simulink library "PhD_Library"  (R2018a)
settings: Solver=VariableStepAuto  StartTime=0.0  StopTime=10.0  RelTol=1e-3
values from neighbouring files (symbols this model uses):
  fn = 60    [Basics_01_Param.m]    (also in FIRs.m = 50; PostSubmission_FreqResp_00_Param.m; XoverRCalc.m)
  Ts_control = 1/20000    (= 5e-05)    [Basics_01_Param.m]    (also in PostSubmission_FreqResp_00_Param.m)
  Ts_PWM = 1/200000    (= 5e-06)    [Basics_01_Param.m]    (also in PostSubmission_FreqResp_00_Param.m)
  Uanp = 1    [Basics_01_Param.m]    (also in PostSubmission_FreqResp_00_Param.m)
undefined symbols (not defined in the file or in its folder): D1, Delta, DiscIntNeverNeededParam, ESS, Iap, PCC, Sn, tctrl, WT
libraries: $bdroot x49, powerlib_meascontrol x39, peTransforms x28, powerlib x18
(part 2 of 3)

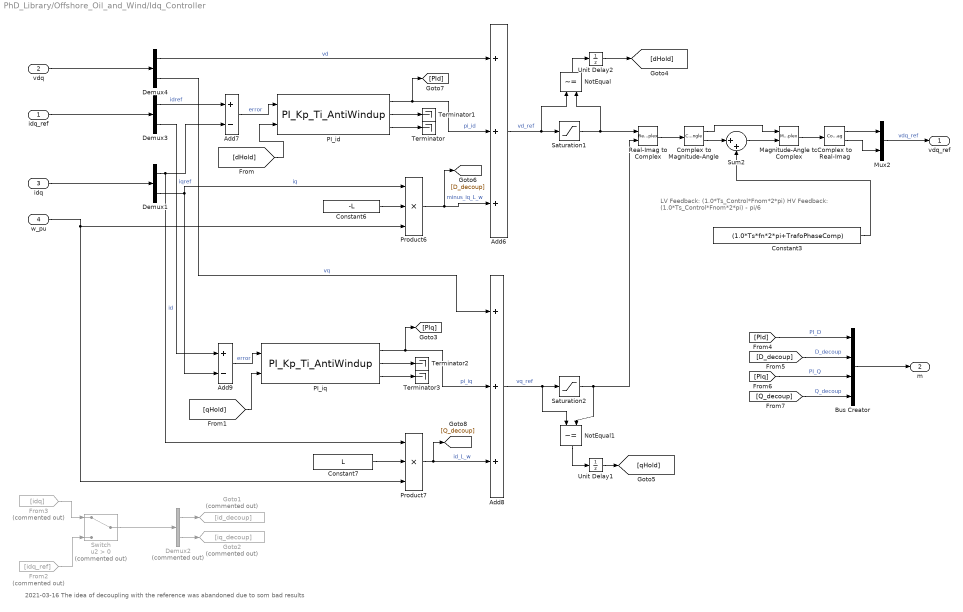
== system PhD_Library/Offshore_Oil_and_Wind/Idq_Controller ==
  note: LV Feedback: (1.0*Ts_Control*Fnom*2*pi)
      | HV Feedback: (1.0*Ts_Control*Fnom*2*pi) - pi/6
  note: 2021-03-16 The idea of decoupling with the reference was abandoned due to som bad results
  idq_ref : Inport
  vdq : Inport  Port=2
  idq : Inport  Port=3
  w_pu : Inport  Port=4
  Add6 : Sum  Inputs=+++
  Add7 : Sum  Inputs=+-
  Add8 : Sum  Inputs=+++
  Add9 : Sum  Inputs=+-
  Bus Creator : BusCreator  Inputs=4
  Complex to Magnitude-Angle : ComplexToMagnitudeAngle
  Complex to Real-Imag : ComplexToRealImag
  Constant3 : Constant  Value=(1.0*Ts*fn*2*pi+TrafoPhaseComp)  SampleTime=Ts
  Constant6 : Constant  Value=-L  SampleTime=Ts_control
  Constant7 : Constant  Value=L  SampleTime=Ts_control
  Demux1 : Demux  Outputs=2
  Demux2 : Demux  Commented=on  Outputs=2
  Demux3 : Demux  Outputs=2
  Demux4 : Demux  Outputs=2
  From2 : From  Commented=on  GotoTag=idq_ref
  From3 : From  Commented=on  GotoTag=idq
  Goto1 : Goto  Commented=on  GotoTag=id_decoup
  Goto2 : Goto  Commented=on  GotoTag=iq_decoup
  Magnitude-Angle to Complex : MagnitudeAngleToComplex
  Mux2 : Mux  Inputs=2
  NotEqual : RelationalOperator  Operator=~=  OutDataTypeStr=boolean  RndMeth=Simplest
  NotEqual1 : RelationalOperator  Operator=~=  OutDataTypeStr=boolean  RndMeth=Simplest
  PI_id : $bdroot/Offshore_Oil_and_Wind/PI_Kp_Ti_AntiWindup  Ts=Ts  Kp=Kp  Ti=Ti  I_ini=I_ini_d  PI_max=PI_max  PI_min=PI_min
  PI_iq : $bdroot/Offshore_Oil_and_Wind/PI_Kp_Ti_AntiWindup  Ts=Ts  Kp=Kp  Ti=Ti  I_ini=I_ini_q  PI_max=PI_max  PI_min=PI_min
  Product6 : Product  Inputs=3  RndMeth=Zero
  Product7 : Product  Inputs=3  RndMeth=Zero
  Real-Imag to Complex : RealImagToComplex
  Saturation1 : Saturate  UpperLimit=PI_max  LowerLimit=PI_min
  Saturation2 : Saturate  UpperLimit=PI_max  LowerLimit=PI_min
  Sum2 : Sum  Inputs=|++
  Switch : Switch  Commented=on  Criteria=u2 > Threshold
  Terminator{,1..3} (4 alike) : Terminator
  Unit Delay1 : UnitDelay  SampleTime=Ts
  Unit Delay2 : UnitDelay  SampleTime=Ts
  vdq_ref : Outport
  m : Outport  Port=2
  wires:
  PI_iq/1 -> [PIq], Add8/2  "pi_iq"
  PI_iq/2 -> Terminator2/1
  PI_id/2 -> Terminator1/1
  w_pu/1 -> Product7/3, Product6/3
  Add9/1 -> PI_iq/1  "error"
  PI_id/1 -> [PId], Add6/2  "pi_id"
  Constant6/1 -> Product6/2
  Constant7/1 -> Product7/2
  Demux1/1 -> Add7/2, Product7/1  "id"
  Product7/1 -> [Q_decoup], Add8/3  "id_L_w"
  Demux4/1 -> Add6/1  "vd"
  Add7/1 -> PI_id/1  "error"
  Demux1/2 -> Product6/1, Add9/2  "iq"
  Product6/1 -> [D_decoup], Add6/3  "minus_iq_L_w"
  PI_iq/3 -> Terminator3/1
  PI_id/3 -> Terminator/1
  Demux4/2 -> Add8/1  "vq"
  Mux2/1 -> vdq_ref/1  "vdq_ref"
  idq/1 -> Demux1/1
  vdq/1 -> Demux4/1
  Add8/1 -> NotEqual1/1, Saturation2/1  "vq_ref"
  Add6/1 -> NotEqual/1, Saturation1/1  "vd_ref"
  Demux2/1 -> Goto1/1
  Demux2/2 -> Goto2/1
  idq_ref/1 -> Demux3/1
  Demux3/1 -> Add7/1  "idref"
  Demux3/2 -> Add9/1  "iqref"
  Switch/1 -> Demux2/1
  From2/1 -> Switch/3
  From3/1 -> Switch/1
  Magnitude-Angle to Complex/1 -> Complex to Real-Imag/1
  Real-Imag to Complex/1 -> Complex to Magnitude-Angle/1
  Complex to Magnitude-Angle/1 -> Magnitude-Angle to Complex/1
  Complex to Magnitude-Angle/2 -> Sum2/1
  Sum2/1 -> Magnitude-Angle to Complex/2
  Constant3/1 -> Sum2/2
  Complex to Real-Imag/1 -> Mux2/1
  Complex to Real-Imag/2 -> Mux2/2
  [PId] -> Bus Creator/1  "PI_D"
  [D_decoup] -> Bus Creator/2  "D_decoup"
  [PIq] -> Bus Creator/3  "PI_Q"
  Bus Creator/1 -> m/1
  [Q_decoup] -> Bus Creator/4  "Q_decoup"
  Saturation1/1 -> NotEqual/2, Real-Imag to Complex/1
  NotEqual/1 -> Unit Delay2/1
  Saturation2/1 -> NotEqual1/2, Real-Imag to Complex/2
  NotEqual1/1 -> Unit Delay1/1
  Unit Delay2/1 -> [dHold]
  Unit Delay1/1 -> [qHold]
  [dHold] -> PI_id/2
  [qHold] -> PI_iq/2

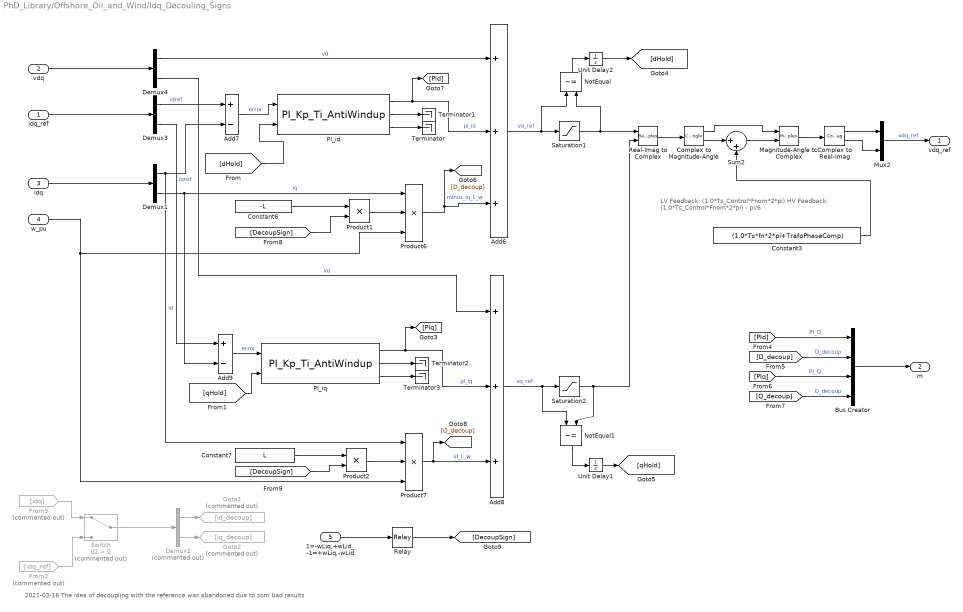
== system PhD_Library/Offshore_Oil_and_Wind/Idq_Decouling_Signs ==
  note: LV Feedback: (1.0*Ts_Control*Fnom*2*pi)
      | HV Feedback: (1.0*Ts_Control*Fnom*2*pi) - pi/6
  note: 2021-03-16 The idea of decoupling with the reference was abandoned due to som bad results
  idq_ref : Inport
  vdq : Inport  Port=2
  idq : Inport  Port=3
  w_pu : Inport  Port=4
  1=-wLiq,+wLid_-1=+wLiq,-wLid : Inport  Port=5
  Add6 : Sum  Inputs=+++
  Add7 : Sum  Inputs=+-
  Add8 : Sum  Inputs=+++
  Add9 : Sum  Inputs=+-
  Bus Creator : BusCreator  Inputs=4
  Complex to Magnitude-Angle : ComplexToMagnitudeAngle
  Complex to Real-Imag : ComplexToRealImag
  Constant3 : Constant  Value=(1.0*Ts*fn*2*pi+TrafoPhaseComp)  SampleTime=Ts
  Constant6 : Constant  Value=-L  SampleTime=Ts_control
  Constant7 : Constant  Value=L  SampleTime=Ts_control
  Demux1 : Demux  Outputs=2
  Demux2 : Demux  Commented=on  Outputs=2
  Demux3 : Demux  Outputs=2
  Demux4 : Demux  Outputs=2
  From2 : From  Commented=on  GotoTag=idq_ref
  From3 : From  Commented=on  GotoTag=idq
  Goto1 : Goto  Commented=on  GotoTag=id_decoup
  Goto2 : Goto  Commented=on  GotoTag=iq_decoup
  Magnitude-Angle to Complex : MagnitudeAngleToComplex
  Mux2 : Mux  Inputs=2
  NotEqual : RelationalOperator  Operator=~=  OutDataTypeStr=boolean  RndMeth=Simplest
  NotEqual1 : RelationalOperator  Operator=~=  OutDataTypeStr=boolean  RndMeth=Simplest
  PI_id : $bdroot/Offshore_Oil_and_Wind/PI_Kp_Ti_AntiWindup  Ts=Ts  Kp=Kp  Ti=Ti  I_ini=I_ini_d  PI_max=PI_max  PI_min=PI_min
  PI_iq : $bdroot/Offshore_Oil_and_Wind/PI_Kp_Ti_AntiWindup  Ts=Ts  Kp=Kp  Ti=Ti  I_ini=I_ini_q  PI_max=PI_max  PI_min=PI_min
  Product1 : Product  RndMeth=Zero
  Product2 : Product  RndMeth=Zero
  Product6 : Product  Inputs=3  RndMeth=Zero
  Product7 : Product  Inputs=3  RndMeth=Zero
  Real-Imag to Complex : RealImagToComplex
  Relay : Relay  OnSwitchValue=0  OffSwitchValue=-0.1  OffOutputValue=-1
  Saturation1 : Saturate  UpperLimit=PI_max  LowerLimit=PI_min
  Saturation2 : Saturate  UpperLimit=PI_max  LowerLimit=PI_min
  Sum2 : Sum  Inputs=|++
  Switch : Switch  Commented=on  Criteria=u2 > Threshold
  Terminator{,1..3} (4 alike) : Terminator
  Unit Delay1 : UnitDelay  SampleTime=Ts
  Unit Delay2 : UnitDelay  SampleTime=Ts
  vdq_ref : Outport
  m : Outport  Port=2
  wires:
  PI_iq/1 -> [PIq], Add8/2  "pi_iq"
  PI_iq/2 -> Terminator2/1
  PI_id/2 -> Terminator1/1
  w_pu/1 -> Product7/3, Product6/3
  Add9/1 -> PI_iq/1  "error"
  PI_id/1 -> [PId], Add6/2  "pi_id"
  Constant6/1 -> Product1/1
  Constant7/1 -> Product2/1
  Demux1/1 -> Add7/2, Product7/1  "id"
  Product7/1 -> [Q_decoup], Add8/3  "id_L_w"
  Demux4/1 -> Add6/1  "vd"
  Add7/1 -> PI_id/1  "error"
  Demux1/2 -> Product6/1, Add9/2  "iq"
  Product6/1 -> [D_decoup], Add6/3  "minus_iq_L_w"
  PI_iq/3 -> Terminator3/1
  PI_id/3 -> Terminator/1
  Demux4/2 -> Add8/1  "vq"
  Mux2/1 -> vdq_ref/1  "vdq_ref"
  idq/1 -> Demux1/1
  vdq/1 -> Demux4/1
  Add8/1 -> NotEqual1/1, Saturation2/1  "vq_ref"
  Add6/1 -> NotEqual/1, Saturation1/1  "vd_ref"
  Demux2/1 -> Goto1/1
  Demux2/2 -> Goto2/1
  idq_ref/1 -> Demux3/1
  Demux3/1 -> Add7/1  "idref"
  Demux3/2 -> Add9/1  "iqref"
  Switch/1 -> Demux2/1
  From2/1 -> Switch/3
  From3/1 -> Switch/1
  Magnitude-Angle to Complex/1 -> Complex to Real-Imag/1
  Real-Imag to Complex/1 -> Complex to Magnitude-Angle/1
  Complex to Magnitude-Angle/1 -> Magnitude-Angle to Complex/1
  Complex to Magnitude-Angle/2 -> Sum2/1
  Sum2/1 -> Magnitude-Angle to Complex/2
  Constant3/1 -> Sum2/2
  Complex to Real-Imag/1 -> Mux2/1
  Complex to Real-Imag/2 -> Mux2/2
  [PId] -> Bus Creator/1  "PI_D"
  [D_decoup] -> Bus Creator/2  "D_decoup"
  [PIq] -> Bus Creator/3  "PI_Q"
  Bus Creator/1 -> m/1
  [Q_decoup] -> Bus Creator/4  "Q_decoup"
  Saturation1/1 -> NotEqual/2, Real-Imag to Complex/1
  NotEqual/1 -> Unit Delay2/1
  Saturation2/1 -> NotEqual1/2, Real-Imag to Complex/2
  NotEqual1/1 -> Unit Delay1/1
  Unit Delay2/1 -> [dHold]
  Unit Delay1/1 -> [qHold]
  [dHold] -> PI_id/2
  [qHold] -> PI_iq/2
  Relay/1 -> [DecoupSign]
  1=-wLiq,+wLid_-1=+wLiq,-wLid/1 -> Relay/1
  [DecoupSign] -> Product1/2
  Product1/1 -> Product6/2
  Product2/1 -> Product7/2
  [DecoupSign] -> Product2/2

== system PhD_Library/Offshore_Oil_and_Wind/LSC_LCL_Trafo ==
  Gates : Inport
  Block_IGBTs : Inport  Port=2
  Open_Close_Breaker : Inport  Port=3
  Bus Creator : BusCreator  Inputs=8
  HV : powerlib/Measurements/Three-Phase V-I Measurement  VoltageMeasurement=phase-to-ground  SetLabelV=off  LabelV=vgrid  Vpu=off  VpuLL=off  CurrentMeasurement=yes  SetLabelI=off  LabelI=igrid  Ipu=off  Pbase=sn  Vbase=uab  OutputType=Complex  PhasorSimulation=off  PSBequivalent=0
  High Res Grounding : powerlib/Elements/Three-Phase Parallel RLC Load  LConnTagsString=A|B|C  Configuration=Y (grounded)  NominalVoltage=Uab  Vabc=[1e3 1e3 1e3]  Vabcp=[1e3 1e3 1e3]  NominalFrequency=fn  UnbalancedPower=off  ActivePower=0.001  InductivePower=0  CapacitivePower=0  Pabc=[10e3 9e3 11e3]  QLabc=[100 90 110]  QCabc=[100 90 110]  Pabcp=[10e3 9e3 11e3]  QLabcp=[100 90 110]  QCabcp=[100 90 110]  Measurements=None  LoadType=constant Z
  INV : powerlib/Measurements/Three-Phase V-I Measurement  VoltageMeasurement=phase-to-ground  SetLabelV=off  LabelV=vconv  Vpu=off  VpuLL=off  CurrentMeasurement=yes  SetLabelI=off  LabelI=iconv  Ipu=off  Pbase=sn  Vbase=uab  OutputType=Complex  PhasorSimulation=off  PSBequivalent=0
  INV_DClink : Subsystem
  LSC : powerlib/Power Electronics/Two-Level Converter  ModelType=Switching devices  Ron=1e-3  Rs=1e6  Cs=inf  Vforward=[ 0, 0 ]  Ron_Diode=1e-3  Rs_Diode=1e6  Cs_Diode=inf  Vf_Diode=1e-3  Rs_CurrentSource=inf
      settings: AttributesFormatString=%<ModelType>  SourceProductName=Simscape Power Systems  SourceProductBaseCode=PS
  LV : powerlib/Measurements/Three-Phase V-I Measurement  VoltageMeasurement=phase-to-ground  SetLabelV=off  LabelV=vgrid  Vpu=off  VpuLL=off  CurrentMeasurement=yes  SetLabelI=off  LabelI=igrid  Ipu=off  Pbase=sn  Vbase=uab  OutputType=Complex  PhasorSimulation=off  PSBequivalent=0
  La_DVR1 : powerlib/Elements/Series RLC Branch  LConnTagsString=__new0  RConnTagsString=__new0  BranchType=RL  Resistance=Rf1  Inductance=Lf1  SetiL0=off  InitialCurrent=0  Capacitance=1.0  Setx0=off  InitialVoltage=0  Measurements=None
  La_DVR2 : powerlib/Elements/Series RLC Branch  LConnTagsString=__new0  RConnTagsString=__new0  BranchType=RL  Resistance=Rf1  Inductance=Lf1  SetiL0=off  InitialCurrent=0  Capacitance=1.0  Setx0=off  InitialVoltage=0  Measurements=None
  La_DVR3 : powerlib/Elements/Series RLC Branch  LConnTagsString=__new0  RConnTagsString=__new0  BranchType=RL  Resistance=Rf1  Inductance=Lf1  SetiL0=off  InitialCurrent=0  Capacitance=1.0  Setx0=off  InitialVoltage=0  Measurements=None
  La_DVR4 : powerlib/Elements/Series RLC Branch  LConnTagsString=__new0  RConnTagsString=__new0  BranchType=RC  Resistance=Rc  Inductance=Lf1  SetiL0=off  InitialCurrent=0  Capacitance=Cf  Setx0=off  InitialVoltage=0  Measurements=None
  La_DVR5 : powerlib/Elements/Series RLC Branch  LConnTagsString=__new0  RConnTagsString=__new0  BranchType=RC  Resistance=Rc  Inductance=Lf1  SetiL0=off  InitialCurrent=0  Capacitance=Cf  Setx0=off  InitialVoltage=0  Measurements=None
  La_DVR6 : powerlib/Elements/Series RLC Branch  LConnTagsString=__new0  RConnTagsString=__new0  BranchType=RC  Resistance=Rc  Inductance=Lf1  SetiL0=off  InitialCurrent=0  Capacitance=Cf  Setx0=off  InitialVoltage=0  Measurements=None
  Three-Phase Transformer (Two Windings) : powerlib/Elements/Three-Phase Transformer (Two Windings)  Winding1Connection=Y  Winding2Connection=Delta (D1)  CoreType=Three-limb core (core-type)  SetSaturation=off  Hysteresis=off  DataFile='hysteresis'  SetInitialFlux=off  Measurements=None  UNITS=pu  NominalPower=[ Sn , fn ]  Winding1=[ Uhv_ab , rf2/2 , lf2/2 ]  Winding2=[ Uab , rf2/2 , lf2/2 ]  Rm=500  Lm=500  L0=0.5  Saturation=[ 0,0 ; 0.0024,1.2 ; 1.0,1.52 ]  InitialFluxes=[0 0 0]  MoreParameters=off  BreakLoop=off  DataType=off  TransfoNumber=1
  Three-Phase Breaker : powerlib/Elements/Three-Phase Breaker  InitialState=open  SwitchA=on  SwitchB=on  SwitchC=on  SwitchTimes="[1/60  5/60]"  External=on  BreakerResistance=0.01  SnubberResistance=1e6  SnubberCapacitance=inf  Measurements=None
  "\tP" : PMIOPort  Side=Left
  M : PMIOPort  Port=2  Side=Left
  A : PMIOPort  Port=3  Side=Right
  B : PMIOPort  Port=4  Side=Right
  C : PMIOPort  Port=5  Side=Right
  m : Outport
  wires:
  HV/2 -> Bus Creator/2  "HV_Iabc"
  LV/1 -> Bus Creator/3  "LV_Vabc"
  INV/1 -> Bus Creator/5  "INV_Vabc"
  INV_DClink/2(Idc) -> Bus Creator/8  "Idc"
  INV/2 -> Bus Creator/6  "INV_Iabc"
  Block_IGBTs/1 -> LSC/2
  INV_DClink/1(Vdc) -> Bus Creator/7  "Vdc"
  HV/1 -> Bus Creator/1  "HV_Vabc"
  LV/2 -> Bus Creator/4  "LV_Iabc"
  Bus Creator/1 -> m/1
  Gates/1 -> LSC/1
  Open_Close_Breaker/1 -> Three-Phase Breaker/1
  connections:
  La_DVR1/LConn1 -- INV/RConn1
  LV/RConn1 -- Three-Phase Transformer (Two Windings)/RConn1 -- High Res Grounding/LConn1
  La_DVR1/RConn1 -- La_DVR4/RConn1 -- LV/LConn1
  LSC/LConn3 -- INV/LConn3
  Three-Phase Transformer (Two Windings)/LConn3 -- HV/LConn3
  LSC/LConn2 -- INV/LConn2
  Three-Phase Transformer (Two Windings)/RConn3 -- LV/RConn3 -- High Res Grounding/LConn3
  La_DVR2/RConn1 -- La_DVR5/RConn1 -- LV/LConn2
  Three-Phase Transformer (Two Windings)/LConn2 -- HV/LConn2
  LSC/RConn2 -- INV_DClink/RConn2
  LSC/LConn1 -- INV/LConn1
  LSC/RConn1 -- INV_DClink/RConn1
  Three-Phase Transformer (Two Windings)/RConn2 -- LV/RConn2 -- High Res Grounding/LConn2
  "\tP"/RConn1 -- INV_DClink/LConn1
  Three-Phase Transformer (Two Windings)/LConn1 -- HV/LConn1
  LV/LConn3 -- La_DVR3/RConn1 -- La_DVR6/RConn1
  La_DVR3/LConn1 -- INV/RConn3
  La_DVR5/LConn1 -- La_DVR6/LConn1 -- La_DVR4/LConn1
  La_DVR2/LConn1 -- INV/RConn2
  INV_DClink/LConn2 -- M/RConn1
  Three-Phase Breaker/LConn2 -- B/RConn1
  Three-Phase Breaker/RConn2 -- HV/RConn2
  HV/RConn3 -- Three-Phase Breaker/RConn3
  Three-Phase Breaker/LConn3 -- C/RConn1
  HV/RConn1 -- Three-Phase Breaker/RConn1
  Three-Phase Breaker/LConn1 -- A/RConn1

== system PhD_Library/Offshore_Oil_and_Wind/PI_Kp_Ti_AntiWindup ==
  note: PI: Kp (s Ti + 1) / (s Ti)
  error : Inport
  Ihold : Inport  Port=2
  Add1 : Sum
  Add9 : Sum
  Constant8 : Constant  Value=0
  Discrete-Time Integrator : DiscreteIntegrator  InitialCondition=I_ini  SampleTime=Ts  LimitOutput=on  UpperSaturationLimit=PI_max  LowerSaturationLimit=PI_min  IgnoreLimit=on  ICPrevOutput=DiscIntNeverNeededParam  ICPrevScaledInput=DiscIntNeverNeededParam
  Gain7 : Gain  Gain=Kp
  Gain9 : Gain  Gain=1/Ti
  NotEqual : RelationalOperator  Operator=~=  OutDataTypeStr=boolean  RndMeth=Simplest
  Saturation1 : Saturate  UpperLimit=PI_max  LowerLimit=PI_min
  Switch : Switch  Criteria=u2 > Threshold
  out : Outport
  Punlim : Outport  Port=2
  I : Outport  Port=3
  wires:
  NotEqual/1 -> [StopInt]
  Saturation1/1 -> out/1, NotEqual/2
  error/1 -> Gain7/1
  Discrete-Time Integrator/1 -> I/1, Add9/2
  Add1/1 -> Switch/2
  Constant8/1 -> Switch/1
  Gain7/1 -> Switch/3, Punlim/1, Add9/1
  Switch/1 -> Gain9/1
  Add9/1 -> NotEqual/1, Saturation1/1
  Gain9/1 -> Discrete-Time Integrator/1
  [StopInt] -> Add1/1
  Ihold/1 -> Add1/2

== system PhD_Library/Offshore_Oil_and_Wind/PLL ==
  vabc : Inport
  PLL (3ph) : powerlib_meascontrol/PLL/PLL (3ph)  Fmin=0.8*fn  Par_Init=[PLL_ini, fn]  ParK=[Kp_pll, Ki_pll, Kd_pll]  TcD=1e-4  MaxRateChangeFreq=fn/5  FilterCutOffFreq=fn/2  Ts=Ts  AGC=on
  Rate Transition1 : RateTransition  OutPortSampleTime=Ts
  Rtot_pu1 : Gain  Gain=-1  SaturateOnIntegerOverflow=on  OutDataTypeStr=Inherit: Same as input  ParamDataTypeStr=Inherit: Same as input
  Rtot_pu3 : Gain  Gain=1/fn  SaturateOnIntegerOverflow=on  OutDataTypeStr=Inherit: Same as input  ParamDataTypeStr=Inherit: Same as input
  f_pu : Outport
  wt : Outport  Port=2
  minus_wt : Outport  Port=3
  wires:
  Rtot_pu3/1 -> f_pu/1
  vabc/1 -> Rate Transition1/1
  Rate Transition1/1 -> PLL (3ph)/1
  PLL (3ph)/2 -> Rtot_pu1/1, wt/1
  PLL (3ph)/1 -> Rtot_pu3/1
  Rtot_pu1/1 -> minus_wt/1

== system PhD_Library/Offshore_Oil_and_Wind/PWM ==
  vdq_abc : Inport
  Enable_abc : Inport  Port=2
  vdq_abc_negwt : Inport  Port=3
  Enable_negwt : Inport  Port=4
  Udc : Inport  Port=5
  wt : Inport  Port=6
  Add : Sum
  Bus Creator : BusCreator  Inputs=4
  Constant1 : Constant  Value=0
  Constant10 : Constant  Value=Uabp
  Constant11 : Constant  Value=0
  Gain : Gain  Gain=Uabp/3^0.5
  Gain1 : Gain  Gain=-1
  Mux1 : Mux  Inputs=[2 1]
  Mux3 : Mux  Inputs=[2 1]
  Overmodulation : powerlib_meascontrol/Pulse & Signal Generators/Overmodulation  OverModType=Third harmonic
      settings: SourceProductName=Simscape Power Systems  SourceProductBaseCode=PS
  PWM Gen : powerlib_meascontrol/Pulse & Signal Generators/PWM Generator (2-Level)  ModulatorType=Three-phase bridge (6 pulses)  ModulatorMode=Unsynchronized  Fc=fsw  Pc=PWM_Ini_Phase  nF=27  MinMax="[ -1  1 ]"  SamplingTechnique=Asymmetrical regular (double edge)  ModulatingSignals=off  m=0.8  Freq=60  Phase=0  Ts=Ts  ShowCarrierOutport=off
      settings: SourceProductName=Simscape Power Systems
  Product1 : Product  Inputs=***
  Product8 : Product  Inputs=*/
  Product9 : Product  Inputs=***
  Rate Transition1 : RateTransition  OutPortSampleTime=Ts
  Rate Transition3 : RateTransition  OutPortSampleTime=Ts
  Rate Transition5 : RateTransition  OutPortSampleTime=Ts
  Relay : Relay  OnSwitchValue=0.6  OffSwitchValue=0.4
  Relay1 : Relay  OnSwitchValue=0.6  OffSwitchValue=0.4
  Saturation : Saturate  UpperLimit=10*Uabp  LowerLimit=0.001*Uabp
  Unit Delay2 : UnitDelay  InitialCondition=Uabp  SampleTime=Ts
  dq0 to abc : powerlib_meascontrol/Transformations/dq0 to abc  Alignment=90 degrees behind phase A axis
  dq0 to abc1 : powerlib_meascontrol/Transformations/dq0 to abc  Alignment=90 degrees behind phase A axis
  pulses : Outport
  Uabcref : Outport  Port=2
  m : Outport  Port=3
  wires:
  dq0 to abc1/1 -> Add/2
  Gain1/1 -> dq0 to abc1/2
  Product1/1 -> Bus Creator/2, dq0 to abc1/1  "vdq0_ref_scaled_NEG"
  vdq_abc_negwt/1 -> Rate Transition1/1
  Constant1/1 -> Mux1/2
  Mux1/1 -> Product1/1
  Product8/1 -> Product1/2, Product9/2
  Rate Transition1/1 -> Mux1/1
  Gain/1 -> Uabcref/1
  Bus Creator/1 -> m/1
  vdq_abc/1 -> Rate Transition3/1
  PWM Gen/1 -> pulses/1
  Udc/1 -> Unit Delay2/1
  Overmodulation/1 -> PWM Gen/1, Bus Creator/4  "uabc_ref"
  Constant10/1 -> Product8/1
  wt/1 -> Rate Transition5/1
  Rate Transition3/1 -> Mux3/1
  Mux3/1 -> Product9/1
  Unit Delay2/1 -> Saturation/1
  Product9/1 -> Bus Creator/1, dq0 to abc/1  "vdq0_ref_scaled_POS"
  Rate Transition5/1 -> dq0 to abc/2, Gain1/1
  Constant11/1 -> Mux3/2
  dq0 to abc/1 -> Add/1
  Enable_abc/1 -> Relay/1
  Relay/1 -> Product9/3
  Enable_negwt/1 -> Relay1/1
  Relay1/1 -> Product1/3
  Add/1 -> Bus Creator/3, Overmodulation/1, Gain/1  "uabc_ref_bef_3rd"
  Saturation/1 -> Product8/2

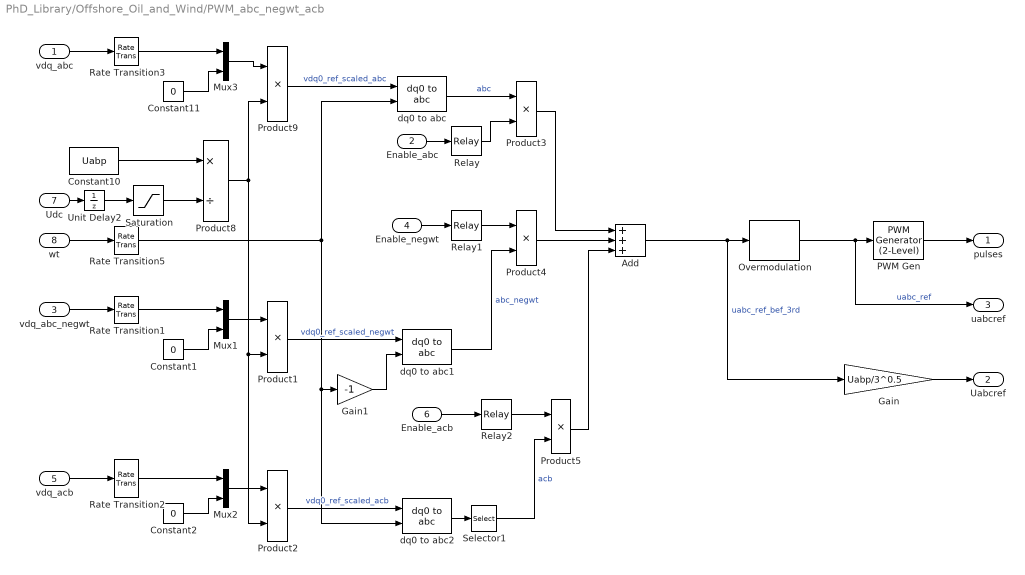
== system PhD_Library/Offshore_Oil_and_Wind/PWM_abc_negwt_acb ==
  vdq_abc : Inport
  Enable_abc : Inport  Port=2
  vdq_abc_negwt : Inport  Port=3
  Enable_negwt : Inport  Port=4
  vdq_acb : Inport  Port=5
  Enable_acb : Inport  Port=6
  Udc : Inport  Port=7
  wt : Inport  Port=8
  Add : Sum  Inputs=+++
  Constant1 : Constant  Value=0
  Constant10 : Constant  Value=Uabp
  Constant11 : Constant  Value=0
  Constant2 : Constant  Value=0
  Gain : Gain  Gain=Uabp/3^0.5
  Gain1 : Gain  Gain=-1
  Mux1 : Mux  Inputs=[2 1]
  Mux2 : Mux  Inputs=[2 1]
  Mux3 : Mux  Inputs=[2 1]
  Overmodulation : powerlib_meascontrol/Pulse & Signal Generators/Overmodulation  OverModType=Third harmonic
      settings: SourceProductName=Simscape Power Systems  SourceProductBaseCode=PS
  PWM Gen : powerlib_meascontrol/Pulse & Signal Generators/PWM Generator (2-Level)  ModulatorType=Three-phase bridge (6 pulses)  ModulatorMode=Unsynchronized  Fc=fsw  Pc=PWM_Ini_Phase  nF=27  MinMax="[ -1  1 ]"  SamplingTechnique=Asymmetrical regular (double edge)  ModulatingSignals=off  m=0.8  Freq=60  Phase=0  Ts=Ts  ShowCarrierOutport=off
      settings: SourceProductName=Simscape Power Systems
  Product{1..5,9} (6 alike) : Product  Inputs=**
  Product8 : Product  Inputs=*/
  Rate Transition{1..3,5} (4 alike) : RateTransition  OutPortSampleTime=Ts
  Relay : Relay  OnSwitchValue=0.6  OffSwitchValue=0.4
  Relay1 : Relay  OnSwitchValue=0.6  OffSwitchValue=0.4
  Relay2 : Relay  OnSwitchValue=0.6  OffSwitchValue=0.4
  Saturation : Saturate  UpperLimit=10*Uabp  LowerLimit=0.001*Uabp
  Selector1 : Selector  InputPortWidth=3  IndexOptions=Index vector (dialog)  Indices=[1 3 2]  OutputSizes=1
  Unit Delay2 : UnitDelay  InitialCondition=Uabp  SampleTime=Ts
  dq0 to abc : powerlib_meascontrol/Transformations/dq0 to abc  Alignment=90 degrees behind phase A axis
  dq0 to abc1 : powerlib_meascontrol/Transformations/dq0 to abc  Alignment=90 degrees behind phase A axis
  dq0 to abc2 : powerlib_meascontrol/Transformations/dq0 to abc  Alignment=90 degrees behind phase A axis
  pulses : Outport
  Uabcref : Outport  Port=2
  uabcref : Outport  Port=3
  wires:
  dq0 to abc1/1 -> Product4/2  "abc_negwt"
  Gain1/1 -> dq0 to abc1/2
  Product1/1 -> dq0 to abc1/1  "vdq0_ref_scaled_negwt"
  vdq_abc_negwt/1 -> Rate Transition1/1
  Constant1/1 -> Mux1/2
  Mux1/1 -> Product1/1
  Rate Transition1/1 -> Mux1/1
  Gain/1 -> Uabcref/1
  vdq_abc/1 -> Rate Transition3/1
  PWM Gen/1 -> pulses/1
  Udc/1 -> Unit Delay2/1
  Overmodulation/1 -> uabcref/1, PWM Gen/1  "uabc_ref"
  Constant10/1 -> Product8/1
  wt/1 -> Rate Transition5/1
  Rate Transition3/1 -> Mux3/1
  Mux3/1 -> Product9/1
  Unit Delay2/1 -> Saturation/1
  Product9/1 -> dq0 to abc/1  "vdq0_ref_scaled_abc"
  Rate Transition5/1 -> dq0 to abc/2, dq0 to abc2/2, Gain1/1
  Constant11/1 -> Mux3/2
  dq0 to abc/1 -> Product3/1  "abc"
  Enable_abc/1 -> Relay/1
  Enable_negwt/1 -> Relay1/1
  Add/1 -> Overmodulation/1, Gain/1  "uabc_ref_bef_3rd"
  Saturation/1 -> Product8/2
  Product8/1 -> Product2/2, Product1/2, Product9/2
  Rate Transition2/1 -> Mux2/1
  vdq_acb/1 -> Rate Transition2/1
  Enable_acb/1 -> Relay2/1
  Mux2/1 -> Product2/1
  Constant2/1 -> Mux2/2
  Product2/1 -> dq0 to abc2/1  "vdq0_ref_scaled_acb"
  dq0 to abc2/1 -> Selector1/1
  Selector1/1 -> Product5/2  "acb"
  Relay/1 -> Product3/2
  Product3/1 -> Add/1
  Product4/1 -> Add/2
  Relay1/1 -> Product4/1
  Relay2/1 -> Product5/1
  Product5/1 -> Add/3

== system PhD_Library/Offshore_Oil_and_Wind/Scaling_and_PWM ==
  vdq_ref_pos : Inport
  Udc : Inport  Port=2
  wt : Inport  Port=3
  vdq_ref_neg : Inport  Port=4
  Bus Creator : BusCreator  Inputs=3
  Constant1 : Constant  Value=0
  Constant10 : Constant  Value=Uabp
  Constant11 : Constant  Value=0
  Gain : Gain  Gain=Uabp/3^0.5
  Gain1 : Gain  Gain=-1
  Mux1 : Mux  Inputs=[2 1]
  Mux3 : Mux  Inputs=[2 1]
  Overmodulation : powerlib_meascontrol/Pulse & Signal Generators/Overmodulation  OverModType=Third harmonic
      settings: SourceProductName=Simscape Power Systems  SourceProductBaseCode=PS
  PWM Gen 1 : powerlib_meascontrol/Pulse & Signal Generators/PWM Generator (2-Level)  ModulatorType=Three-phase bridge (6 pulses)  ModulatorMode=Unsynchronized  Fc=fsw  Pc=PWM_Ini_Phase  nF=27  MinMax="[ -1  1 ]"  SamplingTechnique=Asymmetrical regular (double edge)  ModulatingSignals=off  m=0.8  Freq=60  Phase=0  Ts=Ts  ShowCarrierOutport=off
      settings: SourceProductName=Simscape Power Systems
  Product1 : Product  Inputs=**
  Product8 : Product  Inputs=*/
  Product9 : Product  Inputs=**
  Rate Transition1 : RateTransition  OutPortSampleTime=Ts
  Rate Transition3 : RateTransition  OutPortSampleTime=Ts
  Rate Transition5 : RateTransition  OutPortSampleTime=Ts
  Unit Delay2 : UnitDelay  SampleTime=Ts
  dq0 to abc : powerlib_meascontrol/Transformations/dq0 to abc  Alignment=90 degrees behind phase A axis
  dq0 to abc1 : powerlib_meascontrol/Transformations/dq0 to abc  Alignment=90 degrees behind phase A axis
  pulses : Outport
  Uabcref : Outport  Port=2
  m : Outport  Port=3
  uabc_ref_pos : Outport  Port=4
  uabc_ref_neg : Outport  Port=5
  wires:
  dq0 to abc/1 -> uabc_ref_pos/1, Gain/1, Bus Creator/2, Overmodulation/1  "uabc_ref_bef3rd"
  Constant11/1 -> Mux3/2
  Rate Transition5/1 -> Gain1/1, dq0 to abc/2
  Product9/1 -> Bus Creator/1, dq0 to abc/1  "Vdq0_ref_scaled"
  Unit Delay2/1 -> Product8/2
  Mux3/1 -> Product9/1
  Rate Transition3/1 -> Mux3/1
  wt/1 -> Rate Transition5/1
  Constant10/1 -> Product8/1
  Overmodulation/1 -> Bus Creator/3, PWM Gen 1/1  "uabc_ref"
  Udc/1 -> Unit Delay2/1
  PWM Gen 1/1 -> pulses/1
  vdq_ref_pos/1 -> Rate Transition3/1
  Bus Creator/1 -> m/1
  Gain/1 -> Uabcref/1
  Rate Transition1/1 -> Mux1/1
  Product8/1 -> Product1/2, Product9/2
  Mux1/1 -> Product1/1
  Constant1/1 -> Mux1/2
  vdq_ref_neg/1 -> Rate Transition1/1
  Product1/1 -> dq0 to abc1/1  "Vdq0_ref_scaled"
  Gain1/1 -> dq0 to abc1/2
  dq0 to abc1/1 -> uabc_ref_neg/1

== system PhD_Library/Offshore_Oil_and_Wind/Udc_Controller ==
  vdc : Inport
  Ihold : Inport  Port=2
  Constant1 : Constant
  PI_Kp_Ti_AntiWindup : $bdroot/Offshore_Oil_and_Wind/PI_Kp_Ti_AntiWindup  Ts=Ts  Kp=Kp  Ti=Ti  I_ini=I_ini  PI_max=PI_max  PI_min=PI_min
  Subtract : Sum  Inputs=+-
  Terminator2 : Terminator
  Terminator3 : Terminator
  Unit Delay2 : UnitDelay  SampleTime=Ts
  idref : Outport
  wires:
  PI_Kp_Ti_AntiWindup/2 -> Terminator2/1
  vdc/1 -> Unit Delay2/1  "vdc"
  PI_Kp_Ti_AntiWindup/3 -> Terminator3/1
  Subtract/1 -> PI_Kp_Ti_AntiWindup/1
  Unit Delay2/1 -> Subtract/1
  Constant1/1 -> Subtract/2
  PI_Kp_Ti_AntiWindup/1 -> idref/1  "Idref"
  Ihold/1 -> PI_Kp_Ti_AntiWindup/2

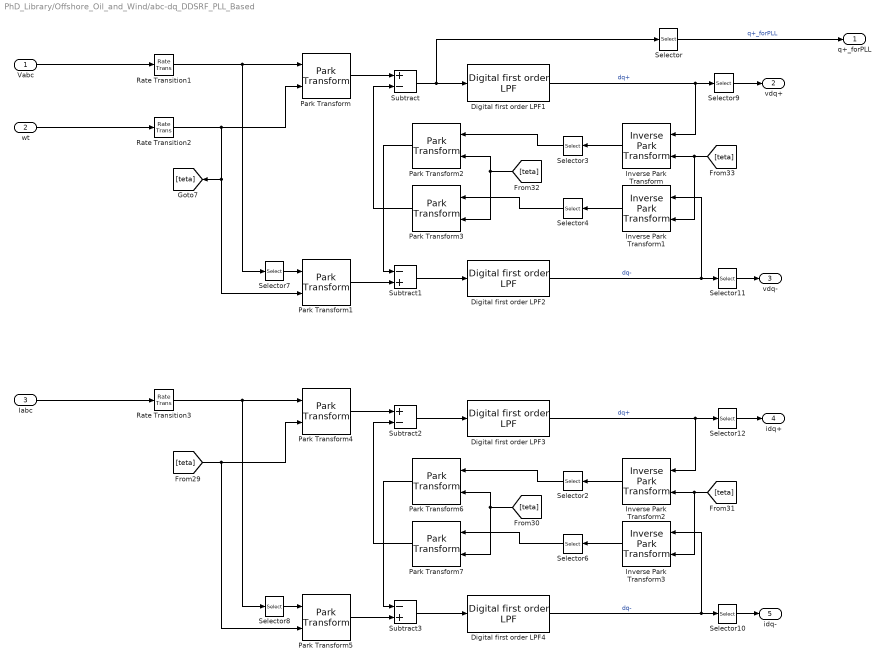
== system PhD_Library/Offshore_Oil_and_Wind/abc-dq_DDSRF_PLL_Based ==
  Vabc : Inport
  wt : Inport  Port=2
  Iabc : Inport  Port=3
  Digital first order LPF{1..4} (4 alike) : $bdroot/Offshore_Oil_and_Wind/Digital first order LPF  Ts=Ts  fcutout=fc
  Inverse Park Transform{,1..3} (4 alike) : peTransforms/Inverse Park Transform  AxisAlignment=Q-axis  PowerInvariant=off
  Park Transform{,1..7} (8 alike) : peTransforms/Park Transform  AxisAlignment=Q-axis  PowerInvariant=off
  Rate Transition1 : RateTransition  OutPortSampleTime=Ts
  Rate Transition2 : RateTransition  OutPortSampleTime=Ts
  Rate Transition3 : RateTransition  OutPortSampleTime=Ts
  Selector : Selector  InputPortWidth=3  IndexOptions=Index vector (dialog)  Indices=2  OutputSizes=1
  Selector{9..12} (4 alike) : Selector  InputPortWidth=3  IndexOptions=Index vector (dialog)  Indices=[1 2]  OutputSizes=1
  Selector{2..4,6..8} (6 alike) : Selector  InputPortWidth=3  IndexOptions=Index vector (dialog)  Indices=[1 3 2]  OutputSizes=1
  Subtract : Sum  Inputs=+-
  Subtract1 : Sum  Inputs=-+
  Subtract2 : Sum  Inputs=+-
  Subtract3 : Sum  Inputs=-+
  q+_forPLL : Outport
  vdq+ : Outport  Port=2
  vdq- : Outport  Port=3
  idq+ : Outport  Port=4
  idq- : Outport  Port=5
  wires:
  Selector/1 -> q+_forPLL/1  "q+_forPLL"
  [teta] -> Inverse Park Transform2/2, Inverse Park Transform3/2
  Rate Transition3/1 -> Selector8/1, Park Transform4/1
  Selector11/1 -> vdq-/1
  Rate Transition1/1 -> Selector7/1, Park Transform/1
  Digital first order LPF4/1 -> Inverse Park Transform3/1, Selector10/1  "dq-"
  Inverse Park Transform3/1 -> Selector6/1
  Rate Transition2/1 -> [teta], Park Transform1/2, Park Transform/2
  Selector4/1 -> Park Transform3/1
  Iabc/1 -> Rate Transition3/1
  [teta] -> Park Transform6/2, Park Transform7/2
  Subtract2/1 -> Digital first order LPF3/1
  Park Transform1/1 -> Subtract1/2
  Selector6/1 -> Park Transform7/1
  Selector8/1 -> Park Transform5/1
  Park Transform7/1 -> Subtract2/2
  Digital first order LPF2/1 -> Selector11/1, Inverse Park Transform1/1  "dq-"
  Selector9/1 -> vdq+/1
  Inverse Park Transform1/1 -> Selector4/1
  Inverse Park Transform2/1 -> Selector2/1
  [teta] -> Park Transform2/2, Park Transform3/2
  Selector10/1 -> idq-/1
  Park Transform2/1 -> Subtract1/1
  Selector2/1 -> Park Transform6/1
  Park Transform5/1 -> Subtract3/2
  Subtract3/1 -> Digital first order LPF4/1
  Subtract1/1 -> Digital first order LPF2/1
  Park Transform/1 -> Subtract/1
  Digital first order LPF3/1 -> Inverse Park Transform2/1, Selector12/1  "dq+"
  Selector12/1 -> idq+/1
  Selector3/1 -> Park Transform2/1
  wt/1 -> Rate Transition2/1
  Park Transform6/1 -> Subtract3/1
  [teta] -> Park Transform5/2, Park Transform4/2
  Park Transform4/1 -> Subtract2/1
  Subtract/1 -> Digital first order LPF1/1, Selector/1
  [teta] -> Inverse Park Transform/2, Inverse Park Transform1/2
  Digital first order LPF1/1 -> Selector9/1, Inverse Park Transform/1  "dq+"
  Vabc/1 -> Rate Transition1/1
  Selector7/1 -> Park Transform1/1
  Inverse Park Transform/1 -> Selector3/1
  Park Transform3/1 -> Subtract/2

== system PhD_Library/Offshore_Oil_and_Wind/abc_dq ==
  vabc : Inport
  iabc : Inport  Port=2
  wt : Inport  Port=3
  Bus Creator : BusCreator  Inputs=4
  Digital first order LPF : $bdroot/Offshore_Oil_and_Wind/Digital first order LPF  Ts=Ts  fcutout=fcutoutv
  Digital first order LPF1 : $bdroot/Offshore_Oil_and_Wind/Digital first order LPF  Ts=Ts  fcutout=fcutouti
  Rate Transition1 : RateTransition  OutPortSampleTime=Ts
  Rate Transition2 : RateTransition  OutPortSampleTime=Ts
  Rate Transition4 : RateTransition  OutPortSampleTime=Ts
  Second-Order Filter1 : powerlib_meascontrol/Filters/Second-Order Filter  FilterType=Bandstop (Notch)  Fo=fn  Zeta=zeta  Ts=Ts  Initialize=off  Vac_Init="[0,  0,  60]"  Vdc_Init=0  PlotResponse=off  FreqRange=[0, 1000, 0.1]
      settings: SourceProductName=Simscape Power Systems  SourceProductBaseCode=PS
  Second-Order Filter5 : powerlib_meascontrol/Filters/Second-Order Filter  FilterType=Bandstop (Notch)  Fo=fn  Zeta=zeta  Ts=Ts  Initialize=off  Vac_Init="[0,  0,  60]"  Vdc_Init=0  PlotResponse=off  FreqRange=[0, 1000, 0.1]
      settings: SourceProductName=Simscape Power Systems  SourceProductBaseCode=PS
  Second-Order Filter Currents : powerlib_meascontrol/Filters/Second-Order Filter  Commented=through  FilterType=Lowpass  Fo=fcutoutv  Zeta=zeta  Ts=Ts  Initialize=off  Vac_Init="[0,  0,  60]"  Vdc_Init=0  PlotResponse=off  FreqRange=[0, 1000, 0.1]
      settings: SourceProductName=Simscape Power Systems  SourceProductBaseCode=PS
  Second-Order Filter Voltages : powerlib_meascontrol/Filters/Second-Order Filter  Commented=through  FilterType=Lowpass  Fo=fcutoutv  Zeta=zeta  Ts=0  Initialize=off  Vac_Init="[0,  0,  60]"  Vdc_Init=0  PlotResponse=off  FreqRange=[0, 1000, 0.1]
      settings: SourceProductName=Simscape Power Systems  SourceProductBaseCode=PS
  Selector4 : Selector  InputPortWidth=3  IndexOptions=Index vector (dialog)  Indices=[1 2]  OutputSizes=1
  Selector5 : Selector  InputPortWidth=3  IndexOptions=Index vector (dialog)  Indices=[1 2]  OutputSizes=1
  abc to dq0 : powerlib_meascontrol/Transformations/abc to dq0  Alignment=90 degrees behind phase A axis
  abc to dq1 : powerlib_meascontrol/Transformations/abc to dq0  Alignment=90 degrees behind phase A axis
  vdq : Outport
  idq : Outport  Port=2
  m : Outport  Port=3
  wires:
  Digital first order LPF1/1 -> Second-Order Filter1/1
  Digital first order LPF/1 -> Second-Order Filter5/1  "vdq"
  abc to dq1/1 -> Selector4/1
  Second-Order Filter1/1 -> Bus Creator/4, idq/1  "idq"
  Selector5/1 -> Digital first order LPF/1, Bus Creator/1  "vdq_unfilt"
  Rate Transition1/1 -> abc to dq0/1
  iabc/1 -> Second-Order Filter Currents/1
  Rate Transition2/1 -> abc to dq1/2, abc to dq0/2
  Selector4/1 -> Bus Creator/2, Digital first order LPF1/1  "idq_unfilt"
  Rate Transition4/1 -> abc to dq1/1
  abc to dq0/1 -> Selector5/1
  Bus Creator/1 -> m/1
  Second-Order Filter5/1 -> vdq/1, Bus Creator/3  "vdq"
  wt/1 -> Rate Transition2/1
  vabc/1 -> Second-Order Filter Voltages/1
  Second-Order Filter Voltages/1 -> Rate Transition1/1
  Second-Order Filter Currents/1 -> Rate Transition4/1

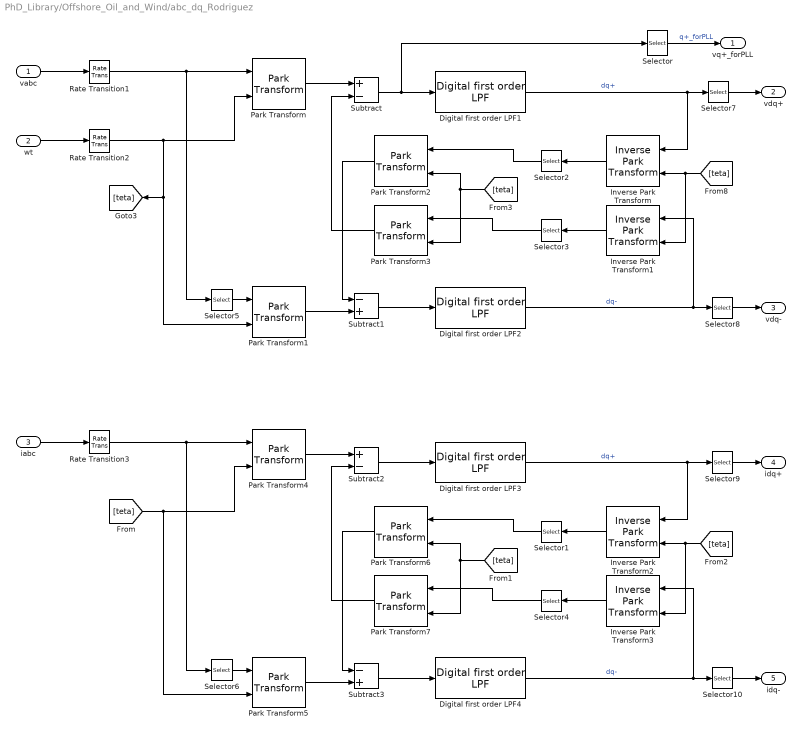
== system PhD_Library/Offshore_Oil_and_Wind/abc_dq_Rodriguez ==
  vabc : Inport
  wt : Inport  Port=2
  iabc : Inport  Port=3
  Digital first order LPF{1..4} (4 alike) : $bdroot/Offshore_Oil_and_Wind/Digital first order LPF  Ts=Ts  fcutout=fcutout
  Inverse Park Transform{,1..3} (4 alike) : peTransforms/Inverse Park Transform  AxisAlignment=Q-axis  PowerInvariant=off
  Park Transform{,1..7} (8 alike) : peTransforms/Park Transform  AxisAlignment=Q-axis  PowerInvariant=off
  Rate Transition1 : RateTransition  OutPortSampleTime=Ts
  Rate Transition2 : RateTransition  OutPortSampleTime=Ts
  Rate Transition3 : RateTransition  OutPortSampleTime=Ts
  Selector : Selector  InputPortWidth=3  IndexOptions=Index vector (dialog)  Indices=2  OutputSizes=1
  Selector{1..6} (6 alike) : Selector  InputPortWidth=3  IndexOptions=Index vector (dialog)  Indices=[1 3 2]  OutputSizes=1
  Selector{7..10} (4 alike) : Selector  InputPortWidth=3  IndexOptions=Index vector (dialog)  Indices=[1 2]  OutputSizes=1
  Subtract : Sum  Inputs=+-
  Subtract1 : Sum  Inputs=-+
  Subtract2 : Sum  Inputs=+-
  Subtract3 : Sum  Inputs=-+
  vq+_forPLL : Outport
  vdq+ : Outport  Port=2
  vdq- : Outport  Port=3
  idq+ : Outport  Port=4
  idq- : Outport  Port=5
  wires:
  Selector/1 -> vq+_forPLL/1  "q+_forPLL"
  Subtract/1 -> Selector/1, Digital first order LPF1/1
  Rate Transition1/1 -> Park Transform/1, Selector5/1
  wt/1 -> Rate Transition2/1
  Park Transform2/1 -> Subtract1/1
  Digital first order LPF1/1 -> Inverse Park Transform/1, Selector7/1  "dq+"
  Rate Transition2/1 -> Park Transform/2, Park Transform1/2, [teta]
  Subtract1/1 -> Digital first order LPF2/1
  Digital first order LPF2/1 -> Inverse Park Transform1/1, Selector8/1  "dq-"
  Park Transform/1 -> Subtract/1
  Park Transform1/1 -> Subtract1/2
  vabc/1 -> Rate Transition1/1
  iabc/1 -> Rate Transition3/1
  [teta] -> Inverse Park Transform1/2, Inverse Park Transform/2
  [teta] -> Park Transform3/2, Park Transform2/2
  Park Transform3/1 -> Subtract/2
  Selector5/1 -> Park Transform1/1
  Inverse Park Transform/1 -> Selector2/1
  Selector2/1 -> Park Transform2/1
  Inverse Park Transform1/1 -> Selector3/1
  Selector3/1 -> Park Transform3/1
  Rate Transition3/1 -> Park Transform4/1, Selector6/1
  [teta] -> Inverse Park Transform3/2, Inverse Park Transform2/2
  Inverse Park Transform2/1 -> Selector1/1
  Inverse Park Transform3/1 -> Selector4/1
  [teta] -> Park Transform7/2, Park Transform6/2
  Park Transform5/1 -> Subtract3/2
  Digital first order LPF3/1 -> Selector9/1, Inverse Park Transform2/1  "dq+"
  Subtract3/1 -> Digital first order LPF4/1
  Selector6/1 -> Park Transform5/1
  [teta] -> Park Transform4/2, Park Transform5/2
  Subtract2/1 -> Digital first order LPF3/1
  Selector4/1 -> Park Transform7/1
  Park Transform7/1 -> Subtract2/2
  Digital first order LPF4/1 -> Selector10/1, Inverse Park Transform3/1  "dq-"
  Park Transform4/1 -> Subtract2/1
  Park Transform6/1 -> Subtract3/1
  Selector1/1 -> Park Transform6/1
  Selector7/1 -> vdq+/1
  Selector8/1 -> vdq-/1
  Selector9/1 -> idq+/1
  Selector10/1 -> idq-/1

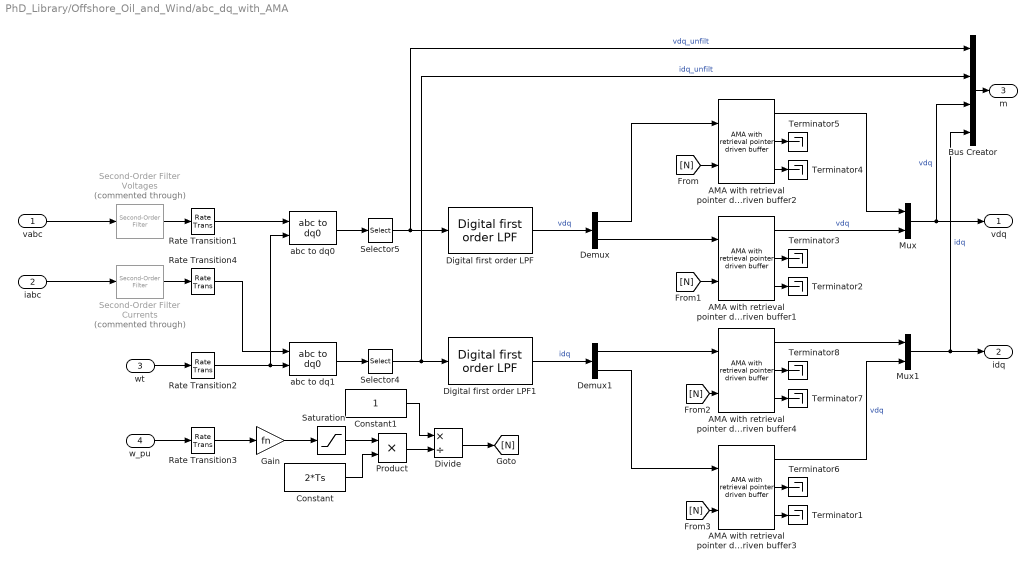
== system PhD_Library/Offshore_Oil_and_Wind/abc_dq_with_AMA ==
  vabc : Inport
  iabc : Inport  Port=2
  wt : Inport  Port=3
  w_pu : Inport  Port=4
  AMA with retrieval pointer driven buffer{1..4} (4 alike) : $bdroot/Adaptive Moving Averages/AMA with retrieval pointer driven buffer  NbSize=1/(2*fmin*Ts)  Ts=Ts
  Bus Creator : BusCreator  Inputs=4
  Constant : Constant  Value=2*Ts
  Constant1 : Constant
  Demux : Demux  Outputs=2
  Demux1 : Demux  Outputs=2
  Digital first order LPF : $bdroot/Offshore_Oil_and_Wind/Digital first order LPF  Ts=Ts  fcutout=fcutoutv
  Digital first order LPF1 : $bdroot/Offshore_Oil_and_Wind/Digital first order LPF  Ts=Ts  fcutout=fcutouti
  Divide : Product  Inputs=*/
  Gain : Gain  Gain=fn
  Mux : Mux  Inputs=2
  Mux1 : Mux  Inputs=2
  Product : Product
  Rate Transition1 : RateTransition  OutPortSampleTime=Ts
  Rate Transition2 : RateTransition  OutPortSampleTime=Ts
  Rate Transition3 : RateTransition  InitialCondition=1  OutPortSampleTime=Ts
  Rate Transition4 : RateTransition  OutPortSampleTime=Ts
  Saturation : Saturate  UpperLimit=fmax  LowerLimit=fmin
  Second-Order Filter Currents : powerlib_meascontrol/Filters/Second-Order Filter  Commented=through  FilterType=Lowpass  Fo=fcutoutv  Zeta=zeta  Ts=Ts  Initialize=off  Vac_Init="[0,  0,  60]"  Vdc_Init=0  PlotResponse=off  FreqRange=[0, 1000, 0.1]
      settings: SourceProductName=Simscape Power Systems  SourceProductBaseCode=PS
  Second-Order Filter Voltages : powerlib_meascontrol/Filters/Second-Order Filter  Commented=through  FilterType=Lowpass  Fo=fcutoutv  Zeta=zeta  Ts=0  Initialize=off  Vac_Init="[0,  0,  60]"  Vdc_Init=0  PlotResponse=off  FreqRange=[0, 1000, 0.1]
      settings: SourceProductName=Simscape Power Systems  SourceProductBaseCode=PS
  Selector4 : Selector  InputPortWidth=3  IndexOptions=Index vector (dialog)  Indices=[1 2]  OutputSizes=1
  Selector5 : Selector  InputPortWidth=3  IndexOptions=Index vector (dialog)  Indices=[1 2]  OutputSizes=1
  Terminator{1..8} (8 alike) : Terminator
  abc to dq0 : powerlib_meascontrol/Transformations/abc to dq0  Alignment=90 degrees behind phase A axis
  abc to dq1 : powerlib_meascontrol/Transformations/abc to dq0  Alignment=90 degrees behind phase A axis
  vdq : Outport
  idq : Outport  Port=2
  m : Outport  Port=3
  wires:
  Digital first order LPF/1 -> Demux/1  "vdq"
  abc to dq1/1 -> Selector4/1
  Mux1/1 -> Bus Creator/4, idq/1  "idq"
  Selector5/1 -> Digital first order LPF/1, Bus Creator/1  "vdq_unfilt"
  Rate Transition1/1 -> abc to dq0/1
  iabc/1 -> Second-Order Filter Currents/1
  Rate Transition2/1 -> abc to dq0/2, abc to dq1/2
  Selector4/1 -> Bus Creator/2, Digital first order LPF1/1  "idq_unfilt"
  Rate Transition4/1 -> abc to dq1/1
  abc to dq0/1 -> Selector5/1
  Bus Creator/1 -> m/1
  Mux/1 -> Bus Creator/3, vdq/1  "vdq"
  wt/1 -> Rate Transition2/1
  vabc/1 -> Second-Order Filter Voltages/1
  Second-Order Filter Voltages/1 -> Rate Transition1/1
  Second-Order Filter Currents/1 -> Rate Transition4/1
  AMA with retrieval pointer driven buffer1/3 -> Terminator2/1
  AMA with retrieval pointer driven buffer1/2 -> Terminator3/1
  w_pu/1 -> Rate Transition3/1
  Rate Transition3/1 -> Gain/1
  Gain/1 -> Saturation/1
  Saturation/1 -> Product/1
  Constant/1 -> Product/2
  Product/1 -> Divide/2
  Constant1/1 -> Divide/1
  Divide/1 -> [N]
  Demux/1 -> AMA with retrieval pointer driven buffer2/1
  Demux/2 -> AMA with retrieval pointer driven buffer1/1
  AMA with retrieval pointer driven buffer2/3 -> Terminator4/1
  AMA with retrieval pointer driven buffer2/2 -> Terminator5/1
  AMA with retrieval pointer driven buffer2/1 -> Mux/1
  AMA with retrieval pointer driven buffer1/1 -> Mux/2  "vdq"
  AMA with retrieval pointer driven buffer3/1 -> Mux1/2  "vdq"
  AMA with retrieval pointer driven buffer4/2 -> Terminator8/1
  Demux1/1 -> AMA with retrieval pointer driven buffer4/1
  Demux1/2 -> AMA with retrieval pointer driven buffer3/1
  AMA with retrieval pointer driven buffer4/3 -> Terminator7/1
  AMA with retrieval pointer driven buffer3/3 -> Terminator1/1
  AMA with retrieval pointer driven buffer4/1 -> Mux1/1
  AMA with retrieval pointer driven buffer3/2 -> Terminator6/1
  Digital first order LPF1/1 -> Demux1/1  "idq"
  [N] -> AMA with retrieval pointer driven buffer2/2
  [N] -> AMA with retrieval pointer driven buffer1/2
  [N] -> AMA with retrieval pointer driven buffer4/2
  [N] -> AMA with retrieval pointer driven buffer3/2

== system PhD_Library/Offshore_Oil_and_Wind/abc_dq_with_PLL ==
  vabc : Inport
  iabc : Inport  Port=2
  Bus Creator : BusCreator  Inputs=4
  PLL (3ph) : powerlib_meascontrol/PLL/PLL (3ph)  Fmin=0.8*fn  Par_Init=[0, fn]  ParK=[Kp_pll, Ki_pll, Kd_pll]  TcD=1e-4  MaxRateChangeFreq=fn/5  FilterCutOffFreq=fn/2  Ts=Ts  AGC=on
  Rate Transition1 : RateTransition  OutPortSampleTime=Ts
  Rate Transition4 : RateTransition  OutPortSampleTime=Ts
  Rtot_pu3 : Gain  Gain=1/fn  SaturateOnIntegerOverflow=on  OutDataTypeStr=Inherit: Same as input  ParamDataTypeStr=Inherit: Same as input
  Second-Order Filter1 : powerlib_meascontrol/Filters/Second-Order Filter  FilterType=Bandstop (Notch)  Fo=fn  Zeta=zeta  Ts=Ts  Initialize=off  Vac_Init="[0,  0,  60]"  Vdc_Init=0  PlotResponse=off  FreqRange=[0, 1000, 0.1]
      settings: SourceProductName=Simscape Power Systems  SourceProductBaseCode=PS
  Second-Order Filter2 : powerlib_meascontrol/Filters/Second-Order Filter  FilterType=Lowpass  Fo=fcutoutv  Zeta=zeta  Ts=Ts  Initialize=off  Vac_Init="[0,  0,  60]"  Vdc_Init=0  PlotResponse=off  FreqRange=[0, 1000, 0.1]
      settings: SourceProductName=Simscape Power Systems  SourceProductBaseCode=PS
  Second-Order Filter3 : powerlib_meascontrol/Filters/Second-Order Filter  FilterType=Lowpass  Fo=fcutouti  Zeta=zeta  Ts=Ts  Initialize=off  Vac_Init="[0,  0,  60]"  Vdc_Init=0  PlotResponse=off  FreqRange=[0, 1000, 0.1]
      settings: SourceProductName=Simscape Power Systems  SourceProductBaseCode=PS
  Second-Order Filter5 : powerlib_meascontrol/Filters/Second-Order Filter  FilterType=Bandstop (Notch)  Fo=fn  Zeta=zeta  Ts=Ts  Initialize=off  Vac_Init="[0,  0,  60]"  Vdc_Init=0  PlotResponse=off  FreqRange=[0, 1000, 0.1]
      settings: SourceProductName=Simscape Power Systems  SourceProductBaseCode=PS
  Selector4 : Selector  InputPortWidth=3  IndexOptions=Index vector (dialog)  Indices=[1 2]  OutputSizes=1
  Selector5 : Selector  InputPortWidth=3  IndexOptions=Index vector (dialog)  Indices=[1 2]  OutputSizes=1
  abc to dq0 : powerlib_meascontrol/Transformations/abc to dq0  Alignment=90 degrees behind phase A axis
  abc to dq1 : powerlib_meascontrol/Transformations/abc to dq0  Alignment=90 degrees behind phase A axis
  vdq : Outport
  idq : Outport  Port=2
  f_pu : Outport  Port=3
  wt : Outport  Port=4
  m : Outport  Port=5
  wires:
  Rtot_pu3/1 -> f_pu/1
  Second-Order Filter3/1 -> Second-Order Filter1/1
  Second-Order Filter2/1 -> Second-Order Filter5/1  "vdq"
  abc to dq1/1 -> Selector4/1
  Second-Order Filter1/1 -> Bus Creator/4, idq/1  "idq"
  vabc/1 -> Rate Transition1/1
  Selector5/1 -> Second-Order Filter2/1, Bus Creator/1  "vdq_unfilt"
  Rate Transition1/1 -> abc to dq0/1, PLL (3ph)/1
  iabc/1 -> Rate Transition4/1
  PLL (3ph)/2 -> wt/1, abc to dq1/2, abc to dq0/2
  Selector4/1 -> Second-Order Filter3/1, Bus Creator/2  "idq_unfilt"
  Rate Transition4/1 -> abc to dq1/1
  abc to dq0/1 -> Selector5/1
  PLL (3ph)/1 -> Rtot_pu3/1
  Bus Creator/1 -> m/1
  Second-Order Filter5/1 -> vdq/1, Bus Creator/3  "vdq"

== system PhD_Library/Offshore_Oil_and_Wind/pqui_Transd_NoZeroSeq ==
  note: Akagi 1984 for p and q
      | calc. without zero seq,
      | factor 3/2 compensates for
      | amplitude invariant
      | Clarke transformation
  Vabc : Inport
  Iabc : Inport  Port=2
  Add3 : Sum  Inputs=+-
  Clarke Transform : peTransforms/Clarke Transform  PowerInvariant=off
  Clarke Transform1 : peTransforms/Clarke Transform  PowerInvariant=off
  Demux1 : Demux  Outputs=2
  Demux4 : Demux  Outputs=2
  Dot Product : DotProduct  InputSameDT=on  OutDataTypeStr=Inherit: Inherit via internal rule
  Gain1 : Gain  Gain=3/2/Sn
  Gain2 : Gain  Gain=3/2/Sn
  Gain3 : Gain  Gain=1/Uanp
  Gain4 : Gain  Gain=1/Iap
  Hypot : Math  Operator=hypot  RndMeth=Zero  SaturateOnIntegerOverflow=on
  Hypot1 : Math  Operator=hypot  RndMeth=Zero  SaturateOnIntegerOverflow=on
  Product3 : Product
  Product4 : Product
  Selector1 : Selector  InputPortWidth=3  IndexOptions=Index vector (dialog)  Indices=[1 2]  OutputSizes=1
  Selector5 : Selector  InputPortWidth=3  IndexOptions=Index vector (dialog)  Indices=[1 2]  OutputSizes=1
  p : Outport
  q : Outport  Port=2
  v : Outport  Port=3
  i : Outport  Port=4
  wires:
  Clarke Transform1/1 -> Selector1/1
  Gain3/1 -> v/1  "v"
  Demux1/2 -> Hypot1/2, Product4/2
  Hypot1/1 -> Gain4/1  "i"
  Selector1/1 -> Demux1/1, Dot Product/2
  Selector5/1 -> Demux4/1, Dot Product/1
  Demux4/1 -> Hypot/1, Product4/1
  Hypot/1 -> Gain3/1  "v"
  Dot Product/1 -> Gain1/1  "p"
  Demux1/1 -> Hypot1/1, Product3/2
  Add3/1 -> Gain2/1  "q"
  Product4/1 -> Add3/2
  Demux4/2 -> Hypot/2, Product3/1
  Vabc/1 -> Clarke Transform/1
  Clarke Transform/1 -> Selector5/1
  Iabc/1 -> Clarke Transform1/1
  Product3/1 -> Add3/1
  Gain1/1 -> p/1  "p"
  Gain4/1 -> i/1  "i"
  Gain2/1 -> q/1  "q"

== system PhD_Library/Offshore_Oil_and_Wind/pqui_Transd_NoZeroSeq_Filter ==
  note: Akagi 1984 for p and q
      | calc. without zero seq,
      | factor 3/2 compensates for
      | amplitude invariant
      | Clarke transformation
  Vabc : Inport
  Iabc : Inport  Port=2
  Add3 : Sum  Inputs=+-
  Clarke Transform : peTransforms/Clarke Transform  PowerInvariant=off
  Clarke Transform1 : peTransforms/Clarke Transform  PowerInvariant=off
  Demux1 : Demux  Outputs=2
  Demux4 : Demux  Outputs=2
  Dot Product : DotProduct  InputSameDT=on  OutDataTypeStr=Inherit: Inherit via internal rule
  Gain1 : Gain  Gain=3/2/Sn
  Gain2 : Gain  Gain=3/2/Sn
  Gain3 : Gain  Gain=1/Uanp
  Gain4 : Gain  Gain=1/Iap
  Hypot : Math  Operator=hypot  RndMeth=Zero  SaturateOnIntegerOverflow=on
  Hypot1 : Math  Operator=hypot  RndMeth=Zero  SaturateOnIntegerOverflow=on
  Product3 : Product
  Product4 : Product
  Rate Transition1 : RateTransition  OutPortSampleTime=Ts
  Rate Transition2 : RateTransition  OutPortSampleTime=Ts
  Second-Order Filter1 : powerlib_meascontrol/Filters/Second-Order Filter  FilterType=Lowpass  Fo=fcutoutvi  Zeta=zeta  Ts=Ts  Initialize=off  Vac_Init="[0,  0,  60]"  Vdc_Init=0  PlotResponse=off  FreqRange=[0, 1000, 0.1]
      settings: SourceProductName=Simscape Power Systems  SourceProductBaseCode=PS
  Second-Order Filter2 : powerlib_meascontrol/Filters/Second-Order Filter  FilterType=Lowpass  Fo=fcutoutvi  Zeta=zeta  Ts=Ts  Initialize=off  Vac_Init="[0,  0,  60]"  Vdc_Init=0  PlotResponse=off  FreqRange=[0, 1000, 0.1]
      settings: SourceProductName=Simscape Power Systems  SourceProductBaseCode=PS
  Second-Order Filter{3,5..6,8} (4 alike) : powerlib_meascontrol/Filters/Second-Order Filter  FilterType=Bandstop (Notch)  Fo=fn  Zeta=zeta  Ts=Ts  Initialize=off  Vac_Init="[0,  0,  60]"  Vdc_Init=0  PlotResponse=off  FreqRange=[0, 1000, 0.1]
      settings: SourceProductName=Simscape Power Systems  SourceProductBaseCode=PS
  Second-Order Filter4 : powerlib_meascontrol/Filters/Second-Order Filter  FilterType=Lowpass  Fo=fcutoutpq  Zeta=zeta  Ts=Ts  Initialize=off  Vac_Init="[0,  0,  60]"  Vdc_Init=0  PlotResponse=off  FreqRange=[0, 1000, 0.1]
      settings: SourceProductName=Simscape Power Systems  SourceProductBaseCode=PS
  Second-Order Filter7 : powerlib_meascontrol/Filters/Second-Order Filter  FilterType=Lowpass  Fo=fcutoutpq  Zeta=zeta  Ts=Ts  Initialize=off  Vac_Init="[0,  0,  60]"  Vdc_Init=0  PlotResponse=off  FreqRange=[0, 1000, 0.1]
      settings: SourceProductName=Simscape Power Systems  SourceProductBaseCode=PS
  Selector1 : Selector  InputPortWidth=3  IndexOptions=Index vector (dialog)  Indices=[1 2]  OutputSizes=1
  Selector5 : Selector  InputPortWidth=3  IndexOptions=Index vector (dialog)  Indices=[1 2]  OutputSizes=1
  p : Outport
  q : Outport  Port=2
  v : Outport  Port=3
  i : Outport  Port=4
  wires:
  Clarke Transform1/1 -> Selector1/1
  Gain3/1 -> Second-Order Filter2/1  "v"
  Demux1/2 -> Hypot1/2, Product4/2
  Hypot1/1 -> Gain4/1  "i"
  Selector1/1 -> Demux1/1, Dot Product/2
  Selector5/1 -> Demux4/1, Dot Product/1
  Demux4/1 -> Hypot/1, Product4/1
  Hypot/1 -> Gain3/1  "v"
  Iabc/1 -> Rate Transition2/1
  Dot Product/1 -> Gain1/1  "p"
  Demux1/1 -> Hypot1/1, Product3/2
  Add3/1 -> Gain2/1  "q"
  Vabc/1 -> Rate Transition1/1
  Product4/1 -> Add3/2
  Demux4/2 -> Hypot/2, Product3/1
  Rate Transition1/1 -> Clarke Transform/1
  Clarke Transform/1 -> Selector5/1
  Rate Transition2/1 -> Clarke Transform1/1
  Product3/1 -> Add3/1
  Gain1/1 -> Second-Order Filter7/1  "p"
  Gain4/1 -> Second-Order Filter1/1  "i"
  Gain2/1 -> Second-Order Filter4/1  "q"
  Second-Order Filter2/1 -> Second-Order Filter5/1
  Second-Order Filter5/1 -> v/1
  Second-Order Filter1/1 -> Second-Order Filter3/1
  Second-Order Filter3/1 -> i/1
  Second-Order Filter4/1 -> Second-Order Filter6/1
  Second-Order Filter6/1 -> q/1
  Second-Order Filter8/1 -> p/1
  Second-Order Filter7/1 -> Second-Order Filter8/1

== system PhD_Library/Offshore_Oil_and_Wind/LSC_LCL_Trafo/INV_DClink ==
  CM : powerlib/Measurements/Current Measurement  PhasorSimulation=off  OutputType=Complex  PSBequivalent=0
  VM1 : powerlib/Measurements/Voltage Measurement  PhasorSimulation=off  OutputType=Complex  PSBequivalent=0
  Pin : PMIOPort  Side=Left
  Min : PMIOPort  Port=2  Side=Left
  Pout : PMIOPort  Port=3  Side=Right
  Mout : PMIOPort  Port=4  Side=Right
  Vdc : Outport
  Idc : Outport  Port=2
  wires:
  CM/1 -> Idc/1
  VM1/1 -> Vdc/1
  connections:
  VM1/LConn2 -- Mout/RConn1 -- Min/RConn1
  VM1/LConn1 -- CM/LConn1 -- Pin/RConn1
  CM/RConn1 -- Pout/RConn1
